simulink model "source_ex"  (R2020a)
settings: Solver=VariableStepAuto  StartTime=0.0  StopTime=10.0  RelTol=1e-3
libraries: simulink x1
settings Model: Creator=lenovo  LastModifiedBy=DELL
settings DataIOCC: ReturnWorkspaceOutputs=off
settings DebuggingCC: ArithmeticOperatorsInVariantConditions=warning
settings SFSimCC: SimUseLocalCustomCode=off  CustomCodeUndefinedFunction=UseInterfaceOnly
settings RTWCC: RTWUseLocalCustomCode=off

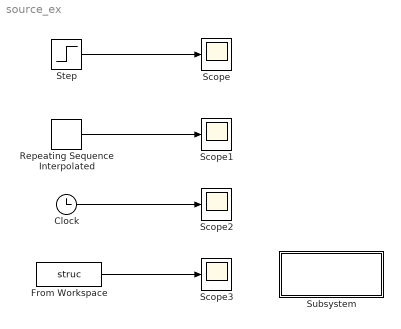
== system source_ex ==
  Clock : Clock
  From Workspace : FromWorkspace  VariableName=struc
  Repeating Sequence Interpolated : simulink/Sources/Repeating Sequence Interpolated  OutValues=[3 1 4 2 1].'  TimeValues=[0 0.1 0.5 0.6 1].'  LookUpMeth=Interpolation-Use End Values  tsamp=0.01  OutMin=[]  OutMax=[]  OutDataTypeStr=double  OutputDataTypeScalingMode=double  OutDataType=fixdt(0,8)  OutScaling=2^-10
  Scope{,1..3} (4 alike) : Scope
  Step : Step  Time=1:5  Before=5:-1:1  After=6:10  SampleTime=0
  Subsystem : Subsystem
      settings: OpenFcn=simin_init;
      mask Display: disp('Init_simin');
  wires:
  Step/1 -> Scope/1
  Repeating Sequence Interpolated/1 -> Scope1/1
  Clock/1 -> Scope2/1
  From Workspace/1 -> Scope3/1

== system source_ex/Subsystem ==
